simulink model "gm_PN_generatorV2_interfaceRX"  (R2020a)
settings: Solver=FixedStepDiscrete  StartTime=0.0  StopTime=20  RelTol=1e-3  EnableMultiTasking=on
undefined symbols (not defined in the file): AXI4, Lite
libraries: axiinterfacelib x3, commfilt2 x2, commchan3 x1, commdigbbndpm3 x1, commseqgen3 x1
settings Model: Creator=juanj  LastModifiedBy=juanj
settings SolverCC: PositivePriorityOrder=on
settings OptimizationCC: BlockReduction=off  ConditionallyExecuteInputs=off  EnhancedBackFolding=on  PassReuseOutputArgsAs=Individual arguments  ZeroExternalMemoryAtStartup=off  ZeroInternalMemoryAtStartup=off  MaxStackSize=64  OptimizeBlockOrder=speed  DifferentSizesBufferReuse=on  OptimizationCustomize=off  EfficientTunableParamExpr=on
settings DebuggingCC: AlgebraicLoopMsg=error  SingleTaskRateTransMsg=error  ParameterTunabilityLossMsg=error
settings HardwareCC: ProdBitPerPointer=32  ProdBitPerSizeT=32  ProdBitPerPtrDiffT=32  ProdLargestAtomicInteger=Long  ProdLargestAtomicFloat=Double  ProdWordSize=32  ProdLongLongMode=on  ProdHWDeviceType=ARM Compatible->ARM Cortex  TargetBitPerPointer=64  TargetBitPerSizeT=64  TargetBitPerPtrDiffT=64  TargetLongLongMode=on  TargetIntDivRoundTo=Zero  TargetEndianess=LittleEndian  TargetWordSize=64  TargetHWDeviceType=Custom Processor->MATLAB Host Computer
settings SFSimCC: MATLABDynamicMemAlloc=off
settings RTWCC: SystemTargetFile=ert.tlc  HardwareBoard=ZedBoard  TemplateMakefile=ert_default_tmf  Toolchain=Linaro AArch32 Linux v6.3.1
settings CodeAppCC: ForceParamTrailComments=on  IgnoreCustomStorageClasses=off  OperatorAnnotations=on  SimulinkDataObjDesc=on  SFDataObjDesc=on  InsertBlockDesc=on

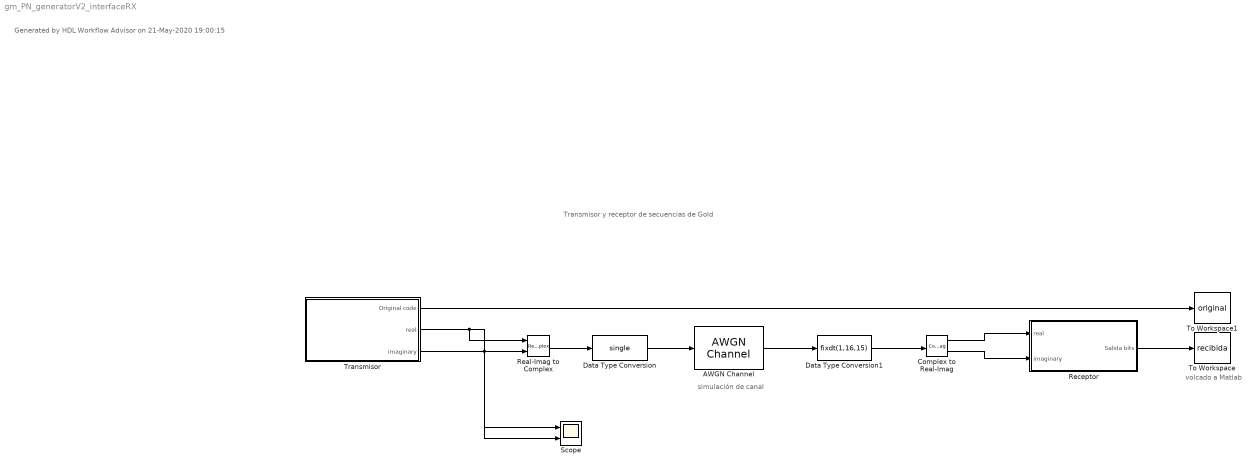
== system gm_PN_generatorV2_interfaceRX ==
  note: Transmisor y receptor de secuencias de Gold
  note: simulación de canal
  note: volcado a Matlab
  note: Generated by HDL Workflow Advisor on 21-May-2020 19:00:15
  AWGN Channel : commchan3/AWGN Channel  InputProcessing=Columns as channels (frame based)  seed=67  noiseMode="Signal to noise ratio  (Es/No)"  EbNodB=10  EsNodB=10  SNRdB=10  bitsPerSym=1  Ps=1  Tsym=0.1  variance=1
  Complex to Real-Imag : ComplexToRealImag
  Data Type Conversion : DataTypeConversion  OutDataTypeStr=single
  Data Type Conversion1 : DataTypeConversion  OutDataTypeStr=fixdt(1,16,15)
  Real-Imag to Complex : RealImagToComplex
  Receptor : Subsystem  TreatAsAtomicUnit=on  mask(AXI4-Lite/AXI4 Interface){}
      mask help:
      | This is an automatically generated subsystem block.
      | This contains the AXI interface blocks that communicate with the Receptor_ip IPCore generated from PN_generatorV2/Receptor subsystem.
      mask Display: disp(sprintf('Xilinx Zynq \nAXI Interface'));
  Scope : Scope  NumInputPorts=2
  To Workspace : ToWorkspace  VariableName=recibida  SampleTime=-1
      settings: Save2DSignal=2-D array (concatenate along first dimension)
  To Workspace1 : ToWorkspace  VariableName=original  SampleTime=-1
      settings: Save2DSignal=2-D array (concatenate along first dimension)
  Transmisor : Subsystem  TreatAsAtomicUnit=on
  wires:
  Transmisor/1(Original code) -> To Workspace1/1
  Data Type Conversion/1 -> AWGN Channel/1
  Data Type Conversion1/1 -> Complex to Real-Imag/1
  AWGN Channel/1 -> Data Type Conversion1/1
  Complex to Real-Imag/2 -> Receptor/2(imaginary)
  Complex to Real-Imag/1 -> Receptor/1(real)
  Transmisor/2(real) -> Real-Imag to Complex/1, Scope/1
  Transmisor/3(imaginary) -> Real-Imag to Complex/2, Scope/2
  Real-Imag to Complex/1 -> Data Type Conversion/1
  Receptor/1(Salida bits) -> To Workspace/1

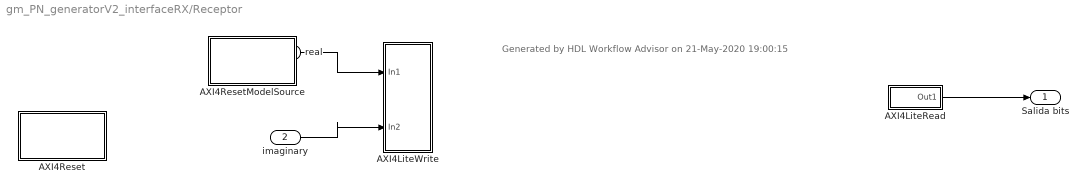
== system gm_PN_generatorV2_interfaceRX/Receptor ==
  note: Generated by HDL Workflow Advisor on 21-May-2020 19:00:15
  real : Inport
  imaginary : Inport  Port=2
  AXI4LiteRead : Subsystem  Priority=10
  AXI4LiteWrite : Subsystem  Priority=1
  AXI4Reset : Subsystem  mask(System Start){ShowInLibBrowser=0}
      mask prompts: ShowInLibBrowser "Simulink:masks:CustCodeMaskParam1_MP"
      settings: CopyFcn=cccopyfcn(gcb)  OpenFcn=ccopenfcn('System Start Function')
      mask Help: eval('feval(''rtwprivate'',''rtwhelpview'',''rtw_sys_start_block'')');
      mask Display: disp('System\nStart');
  AXI4ResetModelSource : Subsystem  mask(Model Source){ShowInLibBrowser=0}
      mask prompts: ShowInLibBrowser "Simulink:masks:CustCodeMaskParam1_MP"
      settings: CopyFcn=cccopyfcn(gcb)  OpenFcn=ccopenfcn('Model Source')
      mask Help: eval('feval(''rtwprivate'',''rtwhelpview'',''rtw_model_source_block'')');
      mask Display: disp('Model\nSource');
  Salida bits : Outport
  wires:
  real/1 -> AXI4LiteWrite/1(In1)
  imaginary/1 -> AXI4LiteWrite/2(In2)
  AXI4LiteRead/1(Out1) -> Salida bits/1

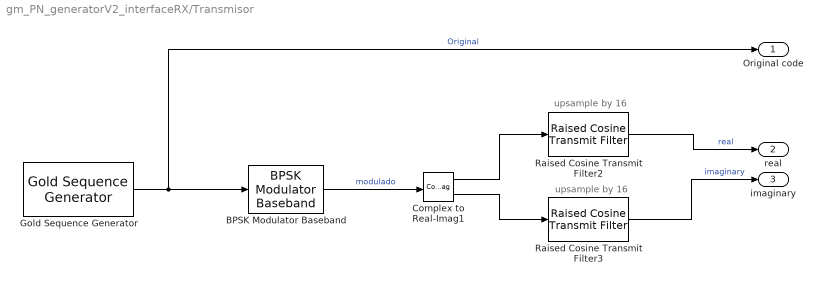
== system gm_PN_generatorV2_interfaceRX/Transmisor ==
  note: upsample by 16
  note: upsample by 16
  BPSK Modulator Baseband : commdigbbndpm3/BPSK Modulator Baseband  Ph=0  outDtype=Fixed-point  outWordLen=16  outUDDataType=sfix(16)  outFracLenMode=Best precision  outFracLen=15  outDataTypeStr=fixdt(1,16)  outLastDataTypeStr=fixdt(1,16)
  Complex to Real-Imag1 : ComplexToRealImag
  Gold Sequence Generator : commseqgen3/Gold Sequence Generator  genPoly1='z^6 + z + 1'  iniState1=[0 1 0 1 0 1]  genPoly2='z^6 + z^5 + z^2 + z + 1'  iniState2=[0 0 0 0 0 1]  index=0  shift=0  outVarSiz=off  maxOutSizeMode=Dialog parameter  maxOutSize=[10 1]  Ts=1/100  sampPerFrame=1  reset=off  outDataType=boolean
      settings: SourceProductBaseCode=CM
  Raised Cosine Transmit Filter2 : commfilt2/Raised Cosine Transmit Filter  filtType=Square root  R=0.5  filtSpan=16  N=16  filterGain=2  RateOptions=Allow multirate processing  framing=Mute  checkCoeff=off  variableName=rcTxFilt2  checkGain=Normalized  sampMode=Mute  saveAsFlag=0  currentFiltSpan=16  D=(16)/2  launchFVT=on  roundingMode=Floor  overflowMode=off  coeffDataTypeStr=Inherit: Same word length as input  coeffMin=[]  coeffMax=[]  coeffLastDataTypeStr=Inherit: Same word length as input  outputMin=[]  outputMax=[]
  Raised Cosine Transmit Filter3 : commfilt2/Raised Cosine Transmit Filter  filtType=Square root  R=0.5  filtSpan=16  N=16  filterGain=2  RateOptions=Allow multirate processing  framing=Mute  checkCoeff=off  variableName=rcTxFilt3  checkGain=Normalized  sampMode=Mute  saveAsFlag=0  currentFiltSpan=16  D=(16)/2  launchFVT=on  roundingMode=Floor  overflowMode=off  coeffDataTypeStr=Inherit: Same word length as input  coeffMin=[]  coeffMax=[]  coeffLastDataTypeStr=Inherit: Same word length as input  outputMin=[]  outputMax=[]
  Original code : Outport
  real : Outport  Port=2
  imaginary : Outport  Port=3
  wires:
  Raised Cosine Transmit Filter2/1 -> real/1  "real"
  Complex to Real-Imag1/2 -> Raised Cosine Transmit Filter3/1
  BPSK Modulator Baseband/1 -> Complex to Real-Imag1/1  "modulado"
  Complex to Real-Imag1/1 -> Raised Cosine Transmit Filter2/1
  Gold Sequence Generator/1 -> BPSK Modulator Baseband/1, Original code/1  "Original"
  Raised Cosine Transmit Filter3/1 -> imaginary/1  "imaginary"

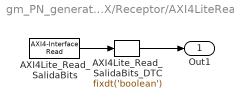
== system gm_PN_generatorV2_interfaceRX/Receptor/AXI4LiteRead ==
  AXI4Lite_Read_SalidaBits : axiinterfacelib/AXI4-Interface Read  Priority=2  AXIInterfaceType=AXI4-Lite  DeviceName=/dev/mwipcore  RegisterOffset=hex2dec('108')  DataLength=1  DataType=uint32  SampleTime=-1  blockPlatform=ZYNQ  SimulateUsing=Interpreted Execution
      settings: SourceProductBaseCode=ECZYNQ7000
  AXI4Lite_Read_SalidaBits_DTC : DataTypeConversion  OutDataTypeStr=fixdt('boolean')  ConvertRealWorld=Stored Integer (SI)
  Out1 : Outport
  wires:
  AXI4Lite_Read_SalidaBits/1 -> AXI4Lite_Read_SalidaBits_DTC/1
  AXI4Lite_Read_SalidaBits_DTC/1 -> Out1/1

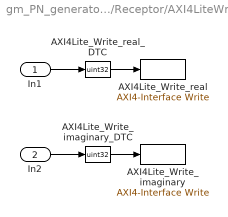
== system gm_PN_generatorV2_interfaceRX/Receptor/AXI4LiteWrite ==
  In1 : Inport
  In2 : Inport  Port=2
  AXI4Lite_Write_imaginary : axiinterfacelib/AXI4-Interface Write  Priority=2  AXIInterfaceType=AXI4-Lite  DeviceName=/dev/mwipcore  RegisterOffset=hex2dec('104')  blockPlatform=ZYNQ  SimulateUsing=Interpreted execution
      settings: SourceProductBaseCode=ECZYNQ7000
  AXI4Lite_Write_imaginary_DTC : DataTypeConversion  OutDataTypeStr=uint32  ConvertRealWorld=Stored Integer (SI)
  AXI4Lite_Write_real : axiinterfacelib/AXI4-Interface Write  Priority=1  AXIInterfaceType=AXI4-Lite  DeviceName=/dev/mwipcore  RegisterOffset=hex2dec('100')  blockPlatform=ZYNQ  SimulateUsing=Interpreted execution
      settings: SourceProductBaseCode=ECZYNQ7000
  AXI4Lite_Write_real_DTC : DataTypeConversion  OutDataTypeStr=uint32  ConvertRealWorld=Stored Integer (SI)
  wires:
  AXI4Lite_Write_imaginary_DTC/1 -> AXI4Lite_Write_imaginary/1
  In1/1 -> AXI4Lite_Write_real_DTC/1
  AXI4Lite_Write_real_DTC/1 -> AXI4Lite_Write_real/1
  In2/1 -> AXI4Lite_Write_imaginary_DTC/1

== system gm_PN_generatorV2_interfaceRX/Receptor/AXI4Reset ==

== system gm_PN_generatorV2_interfaceRX/Receptor/AXI4ResetModelSource ==
